simulink model "Discrete_Model"  (R2020b)
settings: Solver=FixedStepAuto  StartTime=0.0  StopTime=3  FixedStep=0.0001  RelTol=1e-3
values from neighbouring files (symbols this model uses):
  B = 3.4    [nonlinear_quicktest.m]
  cont_den = cont_den_master    [nonlinear_quicktest.m]
  cont_den_master = [0.04052 1 0]    [nonlinear_quicktest.m]
  cont_integrator_discrete = discrete_controller(T_sample, disc_type, [0, 1] , [1, 0] )    [nonlinear_quicktest.m]
  cont_num = cont_num_master    [nonlinear_quicktest.m]
  cont_num_master = [1.517, 3.296, 0.2386]    [nonlinear_quicktest.m]
  Delta = 0.0000079    (= 7.9e-06)    [nonlinear_quicktest.m]
  discrete_constants = zeros(2, 2)    [nonlinear_quicktest.m]
  F_lead_param = -1/(alpha_lead_param*T_lead_param)    [nonlinear_quicktest.m]
  G_lead_param = 1    [nonlinear_quicktest.m]
  H_lead_param = k_lead_param/alpha_lead_param*(1/T_lead_param-1/(alpha_lead_param*T_lead_param))    [nonlinear_quicktest.m]
  J_eq = J_1 + n_1^2 *(J_2 + M_3*r_3^2)    (= 2.88733377778e-05)    [nonlinear_quicktest.m]
  k_i = 0.2386    [nonlinear_quicktest.m]
  k_p = 3.296    [nonlinear_quicktest.m]
  K_tau = 42e-3    (= 0.042)    [nonlinear_quicktest.m]
  L_lead_param = k_lead_param/alpha_lead_param    [nonlinear_quicktest.m]
  M_lead_param = 1/L_lead_param    [nonlinear_quicktest.m]    (also in span_optimering_quicker.m = corrections_faktor(i))
  n_1 = 1/3    (= 0.333333333333)    [nonlinear_quicktest.m]
  r_3 = 0.0127    [nonlinear_quicktest.m]
  step_size = step_size_array(j)    [main.m]    (also in nonlinear_quicktest.m = 1; span_optimering_quicker.m = 1)
  T_sample = 0.001    [main.m]    (also in nonlinear_quicktest.m)
  T_t = (k_p/k_i)/10    (= 1.38139145013)    [nonlinear_quicktest.m]
undefined symbols (not defined in the file or in its folder): CoulombAndViscousFriction, CurrentOffset, discrete_controller_pid, j, SignOfVelocity
settings Model: EnablePacing=on  PacingRate=0.001000  Creator=jonas  LastModifiedBy=Bens PC

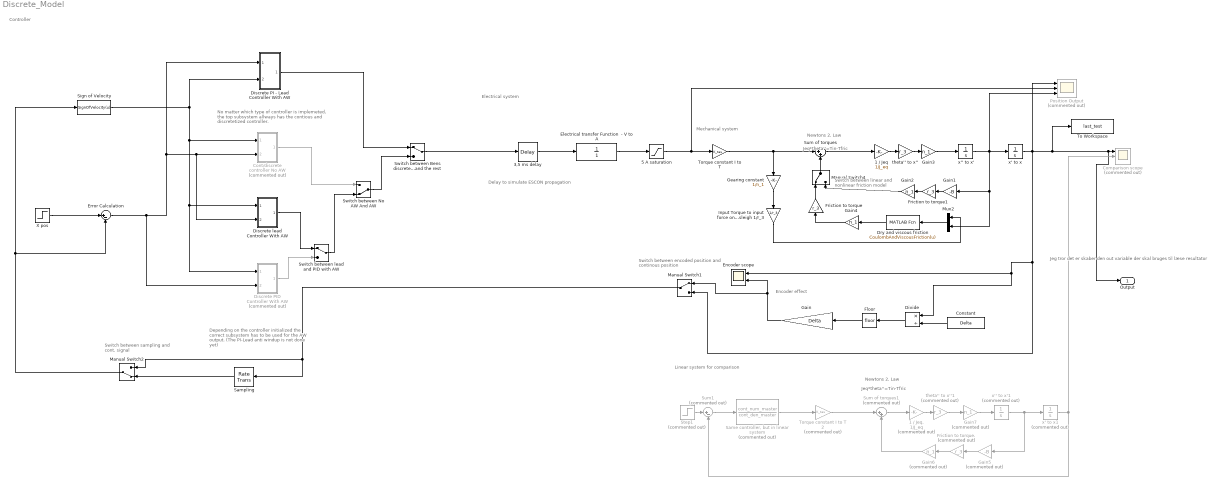
== system Discrete_Model ==
  note: Jeg tror det er skaber den out variable der skal bruges til læse resultator
  note: No matter which type of controller is implemeted,
      | the top subsystem allways has the contious and
      | discretetized controller.
  note: Depending on the controller initialized
      | the correct subsystem has to be used
      | for the AW output. (The PI-Lead anti windup
      | is not done yet)
  note: Controller
  note: Linear system for comparison
  note: Switch between linear
      | and nonlinear friction model
  note: Delay to simulate ESCON propagation
  note: Switch between sampling
      | and cont. signal
  note: Electrical system
  note: Switch between encoded position and
      | continous position
  note: Newtons 2. Law
  note: Mechanical system
  note: Encoder effect
  note: Jeq*theta''=Tin-Tfric
  note: Newtons 2. Law
  note: Jeq*theta''=Tin-Tfric
  1 / Jeq : Gain  Gain=1/J_eq
  1 / Jeq. : Gain  Commented=on  Gain=1/J_eq
  3,5 ms delay : TransportDelay  DelayTime=0.0035
  5 A saturation : Saturate  UpperLimit=5  LowerLimit=-5
  Comparison scope : Scope  Commented=on  NumInputPorts=3
  Constant : Constant  Value=Delta
  Cont/discrete controller No AW : Subsystem  Commented=on
  Discrete PI - Lead Controller With AW : Subsystem
  Discrete PID Controller With AW : Subsystem  Commented=on
  Discrete lead Controller With AW : Subsystem
  Divide : Product  Inputs=*/
  Dry and viscous friction : MATLABFcn  MATLABFcn=CoulombAndViscousFriction(u)  OutputDimensions=1
  Electrical transfer Function  - V to A : TransferFcn  Denominator=[1]
  Encoder scope : Scope  NumInputPorts=2
  Error Calculation : Sum  Inputs=|+-
  Floor : Rounding
  Friction to torque : Gain  Gain=r_3
  Friction to torque. : Gain  Commented=on  Gain=r_3
  Friction to torque1 : Gain  Gain=r_3
  Gain : Gain  Gain=Delta
  Gain1 : Gain  Gain=-B
  Gain2 : Gain  Gain=n_1
  Gain3 : Gain  Gain=n_1
  Gain4 : Gain  Gain=n_1
  Gain5 : Gain  Commented=on  Gain=-B
  Gain6 : Gain  Commented=on  Gain=n_1
  Gain7 : Gain  Commented=on  Gain=n_1
  Gearing constant : Gain  Gain=1/n_1
  Input Torque to input force on sleigh 1/r_3 : Gain  Gain=1/r_3
  Manual Switch1 : ManualSwitch
  Manual Switch2 : ManualSwitch  CurrentSetting=0
  Manual Switch4 : ManualSwitch
  Mux2 : Mux  Inputs=2
  Position Output : Scope  Commented=on  NumInputPorts=3
  "Same controller, but in linear system" : TransferFcn  Commented=on  Numerator=cont_num_master  Denominator=cont_den_master
  "Sampling " : RateTransition  OutPortSampleTime=T_sample
  Sign of Velocity : MATLABFcn  MATLABFcn=SignOfVelocity(u)  OutputDimensions=1
  Step1 : Step  Commented=on  Time=0  After=step_size(j)  SampleTime=0
  Sum of torques : Sum  Inputs=|++
  Sum of torques1 : Sum  Commented=on  Inputs=|++
  Sum1 : Sum  Commented=on  Inputs=|+-
  Switch between Bens discrete PI-Lead AW and the rest : ManualSwitch
  Switch between No AW And AW : ManualSwitch  CurrentSetting=0
  Switch between lead and PID with AW : ManualSwitch
  To Workspace : ToWorkspace  VariableName=last_test  SampleTime=-1
  "Torque constant I to T " : Gain  Gain=K_tau
  Torque constant I to T 2 : Gain  Commented=on  Gain=K_tau
  X pos : Step  Time=0  After=step_size  SampleTime=0
  theta'' to x'' : Gain  Gain=r_3
  theta'' to x''1 : Gain  Commented=on  Gain=r_3
  x' to x : Integrator
  x' to x1 : Integrator  Commented=on
  x'' to x' : Integrator
  x'' to x'1 : Integrator  Commented=on
  Output : Outport
  wires:
  Sum of torques/1 -> 1 / Jeq/1
  theta'' to x''/1 -> Gain3/1
  x'' to x'/1 -> Position Output/3, Gain1/1, Mux2/2, x' to x/1
  Electrical transfer Function  - V to A/1 -> 5 A saturation/1
  Input Torque to input force on sleigh 1/r_3/1 -> Mux2/1
  Mux2/1 -> Dry and viscous friction/1
  5 A saturation/1 -> Position Output/2, "Torque constant I to T "/1
  Gain/1 -> Encoder scope/2, Manual Switch1/1
  Floor/1 -> Gain/1
  Constant/1 -> Divide/2
  Divide/1 -> Floor/1
  Manual Switch1/1 -> "Sampling "/1, Manual Switch2/1
  "Sampling "/1 -> Manual Switch2/2
  Dry and viscous friction/1 -> Gain4/1
  3,5 ms delay/1 -> Electrical transfer Function  - V to A/1
  1 / Jeq/1 -> theta'' to x''/1
  Manual Switch4/1 -> Sum of torques/2
  Friction to torque/1 -> Manual Switch4/1
  Gain1/1 -> Friction to torque1/1
  Friction to torque1/1 -> Gain2/1
  "Torque constant I to T "/1 -> Sum of torques/1, Gearing constant/1
  Gearing constant/1 -> Input Torque to input force on sleigh 1/r_3/1
  Gain2/1 -> Manual Switch4/2
  Gain3/1 -> x'' to x'/1
  Gain4/1 -> Friction to torque/1
  Friction to torque./1 -> Gain6/1
  Gain7/1 -> x'' to x'1/1
  Gain5/1 -> Friction to torque./1
  x'' to x'1/1 -> Gain5/1, x' to x1/1
  Gain6/1 -> Sum of torques1/2
  1 / Jeq./1 -> theta'' to x''1/1
  Sum of torques1/1 -> 1 / Jeq./1
  Sum1/1 -> "Same controller, but in linear system"/1
  Step1/1 -> Sum1/1
  Torque constant I to T 2/1 -> Sum of torques1/1
  x' to x/1 -> Position Output/1, To Workspace/1, Output/1, Comparison scope/1, Divide/1, Encoder scope/1, Manual Switch1/2
  x' to x1/1 -> Comparison scope/2, Sum1/2
  "Same controller, but in linear system"/1 -> Torque constant I to T 2/1
  theta'' to x''1/1 -> Gain7/1
  Sign of Velocity/1 -> Discrete PI - Lead Controller With AW/2(Sign of velocity in), Discrete PID Controller With AW/1(In1), Discrete lead Controller With AW/1(Sign of velocity in), Cont/discrete controller No AW/1(In1)
  Cont/discrete controller No AW/1(Out1) -> Switch between No AW And AW/1
  Discrete lead Controller With AW/1(Out1) -> Switch between lead and PID with AW/1
  Discrete PID Controller With AW/1(Out1) -> Switch between lead and PID with AW/2
  Switch between lead and PID with AW/1 -> Switch between No AW And AW/2
  Manual Switch2/1 -> Sign of Velocity/1, Error Calculation/2
  Discrete PI - Lead Controller With AW/1(Out3) -> Switch between Bens discrete PI-Lead AW and the rest/1
  Switch between No AW And AW/1 -> Switch between Bens discrete PI-Lead AW and the rest/2
  Switch between Bens discrete PI-Lead AW and the rest/1 -> 3,5 ms delay/1
  X pos/1 -> Error Calculation/1
  Error Calculation/1 -> Discrete PID Controller With AW/2(In2), Discrete PI - Lead Controller With AW/1(Error in), Discrete lead Controller With AW/2(Error in), Cont/discrete controller No AW/2(In2)

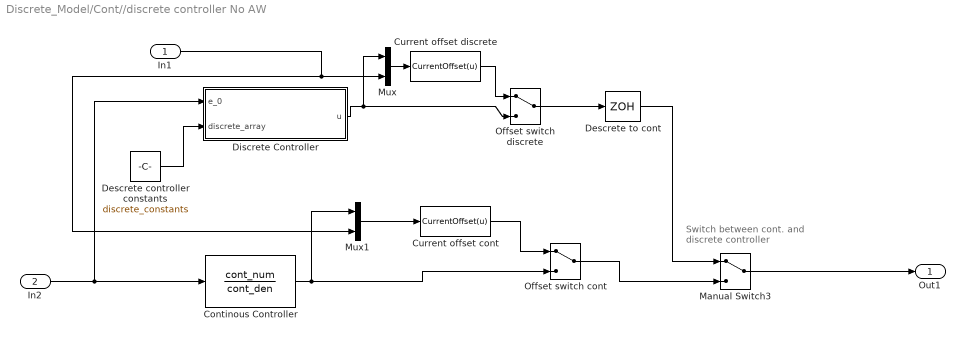
== system Discrete_Model/Cont//discrete controller No AW ==
  note: Switch between cont.
      | and discrete controller
  In1 : Inport
  In2 : Inport  Port=2
  Continous Controller : TransferFcn  Numerator=cont_num  Denominator=cont_den
  Current offset cont : MATLABFcn  MATLABFcn=CurrentOffset(u)  OutputDimensions=1
  Current offset discrete : MATLABFcn  MATLABFcn=CurrentOffset(u)  OutputDimensions=1
  Descrete controller constants : Constant  Value=discrete_constants
  Descrete to cont : ZeroOrderHold  SampleTime=T_sample
  Discrete Controller : MATLAB Function  TreatAsAtomicUnit=on
  Manual Switch3 : ManualSwitch
  Mux : Mux  Inputs=2
  Mux1 : Mux  Inputs=2
  Offset switch cont : ManualSwitch
  Offset switch discrete : ManualSwitch
  Out1 : Outport
  wires:
  Manual Switch3/1 -> Out1/1
  In1/1 -> Mux/2, Mux1/2
  In2/1 -> Continous Controller/1, Discrete Controller/1(e_0)
  Current offset discrete/1 -> Offset switch discrete/1
  Descrete to cont/1 -> Manual Switch3/1
  Offset switch discrete/1 -> Descrete to cont/1
  Offset switch cont/1 -> Manual Switch3/2
  Discrete Controller/1(u) -> Offset switch discrete/2, Mux/1
  Mux/1 -> Current offset discrete/1
  Descrete controller constants/1 -> Discrete Controller/2(discrete_array)
  Mux1/1 -> Current offset cont/1
  Continous Controller/1 -> Mux1/1, Offset switch cont/2
  Current offset cont/1 -> Offset switch cont/1

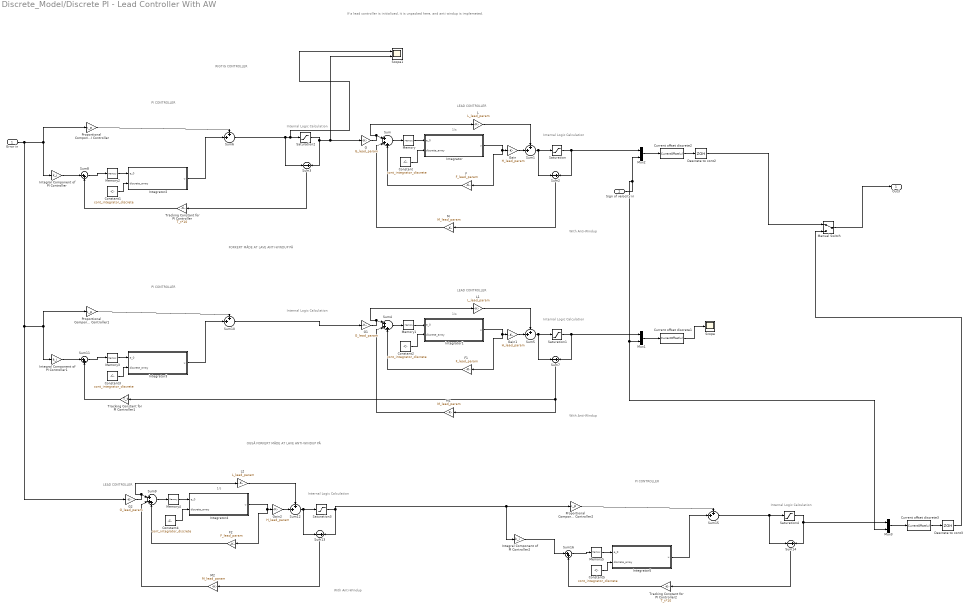
== system Discrete_Model/Discrete PI - Lead Controller With AW ==
  note: RIGTIG CONTROLLER
  note: Internal Logic Calculation
  note: LEAD CONTROLLER
  note: With Anti-Windup
  note: 1/s
  note: If a lead controller is initialized, it is unpacked here, and anti windup is implemeted.
  note: PI CONTROLLER
  note: Internal Logic Calculation
  note: Internal Logic Calculation
  note: LEAD CONTROLLER
  note: With Anti-Windup
  note: 1/s
  note: PI CONTROLLER
  note: Internal Logic Calculation
  note: Internal Logic Calculation
  note: LEAD CONTROLLER
  note: With Anti-Windup
  note: 1/s
  note: PI CONTROLLER
  note: Internal Logic Calculation
  note: FORKERT MÅDE AT LAVE ANTI-WINDUP PÅ
  note: OGSÅ FORKERT MÅDE AT LAVE ANTI-WINDUP PÅ
  Error in : Inport
  Sign of velocity in : Inport  Port=2
  Constant{,1..5} (6 alike) : Constant  Value=cont_integrator_discrete
  Current offset discrete1 : MATLABFcn  MATLABFcn=CurrentOffset(u)  OutputDimensions=1
  Current offset discrete2 : MATLABFcn  MATLABFcn=CurrentOffset(u)  OutputDimensions=1
  Current offset discrete3 : MATLABFcn  MATLABFcn=CurrentOffset(u)  OutputDimensions=1
  Descrete to cont2 : ZeroOrderHold  SampleTime=T_sample
  Descrete to cont3 : ZeroOrderHold  SampleTime=T_sample
  F : Gain  Gain=F_lead_param
  F1 : Gain  Gain=F_lead_param
  F2 : Gain  Gain=F_lead_param
  G : Gain  Gain=G_lead_param
  G1 : Gain  Gain=G_lead_param
  G2 : Gain  Gain=G_lead_param
  Gain : Gain  Gain=H_lead_param
  Gain1 : Gain  Gain=H_lead_param
  Gain2 : Gain  Gain=H_lead_param
  Integral Component of PI Controller : Gain  Gain=k_i
  Integral Component of PI Controller1 : Gain  Gain=k_i
  Integral Component of PI Controller2 : Gain  Gain=k_i
  Integrator : MATLAB Function  TreatAsAtomicUnit=on
  Integrator1 : MATLAB Function  TreatAsAtomicUnit=on
  Integrator2 : MATLAB Function  TreatAsAtomicUnit=on
  Integrator3 : MATLAB Function  TreatAsAtomicUnit=on
  Integrator4 : MATLAB Function  TreatAsAtomicUnit=on
  Integrator5 : MATLAB Function  TreatAsAtomicUnit=on
  L : Gain  Gain=L_lead_param
  L1 : Gain  Gain=L_lead_param
  L2 : Gain  Gain=L_lead_param
  M : Gain  Gain=M_lead_param
  M1 : Gain  Gain=M_lead_param
  M2 : Gain  Gain=M_lead_param
  Manual Switch : ManualSwitch
  Memory{,1..5} (6 alike) : Memory
  Mux1 : Mux  Inputs=2
  Mux2 : Mux  Inputs=2
  Mux3 : Mux  Inputs=2
  Proportional Component of PI Controller : Gain  Gain=k_p
  Proportional Component of PI Controller1 : Gain  Gain=k_p
  Proportional Component of PI Controller2 : Gain  Gain=k_p
  Saturation{,1..4} (5 alike) : Saturate  UpperLimit=5  LowerLimit=-5
  Scope : Scope
  Scope1 : Scope  NumInputPorts=2
  Sum : Sum  Inputs=|+++
  Sum{1,5..6,10,12,15} (6 alike) : Sum  Inputs=++|
  Sum11 : Sum  Inputs=|++
  Sum{2..3,7,13..14} (5 alike) : Sum  Inputs=-+
  Sum16 : Sum  Inputs=|++
  Sum4 : Sum  Inputs=|+++
  Sum8 : Sum  Inputs=|++
  Sum9 : Sum  Inputs=|+++
  Tracking Constant for PI Controller : Gain  Gain=T_t*10
  Tracking Constant for PI Controller1 : Gain  Gain=T_t
  Tracking Constant for PI Controller2 : Gain  Gain=T_t*10
  Out3 : Outport
  wires:
  Mux2/1 -> Current offset discrete2/1
  Current offset discrete2/1 -> Descrete to cont2/1
  Sign of velocity in/1 -> Mux3/2, Mux1/2, Mux2/2
  Sum/1 -> Memory/1
  Memory/1 -> Integrator/1(e_0)
  Saturation/1 -> Mux2/1, Sum2/2
  Constant/1 -> Integrator/2(discrete_array)
  Sum2/1 -> M/1
  M/1 -> Sum/2
  L/1 -> Sum1/1
  Sum1/1 -> Saturation/1, Sum2/1
  G/1 -> L/1, Sum/1
  Integrator/1(u) -> F/1, Gain/1
  F/1 -> Sum/3
  Gain/1 -> Sum1/2
  Saturation2/1 -> Sum3/2, Scope1/2, G/1
  Memory2/1 -> Integrator2/1(e_0)
  Integral Component of PI Controller/1 -> Sum8/1
  Sum8/1 -> Memory2/1
  Constant1/1 -> Integrator2/2(discrete_array)
  Proportional Component of PI Controller/1 -> Sum6/1
  Tracking Constant for PI Controller/1 -> Sum8/2
  Integrator2/1(u) -> Sum6/2
  Sum6/1 -> Scope1/1, Saturation2/1, Sum3/1
  Sum3/1 -> Tracking Constant for PI Controller/1
  Sum7/1 -> M1/1, Tracking Constant for PI Controller1/1
  Integrator3/1(u) -> Sum10/2
  Tracking Constant for PI Controller1/1 -> Sum11/2
  Proportional Component of PI Controller1/1 -> Sum10/1
  Constant3/1 -> Integrator3/2(discrete_array)
  Sum11/1 -> Memory3/1
  Integral Component of PI Controller1/1 -> Sum11/1
  Memory3/1 -> Integrator3/1(e_0)
  Sum10/1 -> G1/1
  Error in/1 -> Proportional Component of PI Controller/1, Integral Component of PI Controller/1, G2/1, Integral Component of PI Controller1/1, Proportional Component of PI Controller1/1
  Gain1/1 -> Sum5/2
  F1/1 -> Sum4/3
  Integrator1/1(u) -> Gain1/1, F1/1
  G1/1 -> Sum4/1, L1/1
  Sum5/1 -> Sum7/1, Saturation1/1
  L1/1 -> Sum5/1
  M1/1 -> Sum4/2
  Constant2/1 -> Integrator1/2(discrete_array)
  Saturation1/1 -> Sum7/2, Mux1/1
  Memory1/1 -> Integrator1/1(e_0)
  Sum4/1 -> Memory1/1
  Mux1/1 -> Current offset discrete1/1
  Descrete to cont2/1 -> Manual Switch/1
  Manual Switch/1 -> Out3/1
  Saturation3/1 -> Integral Component of PI Controller2/1, Proportional Component of PI Controller2/1, Sum13/2
  Sum14/1 -> Tracking Constant for PI Controller2/1
  Sum15/1 -> Sum14/1, Saturation4/1
  Integrator5/1(u) -> Sum15/2
  Tracking Constant for PI Controller2/1 -> Sum16/2
  Proportional Component of PI Controller2/1 -> Sum15/1
  Constant5/1 -> Integrator5/2(discrete_array)
  Sum16/1 -> Memory5/1
  Integral Component of PI Controller2/1 -> Sum16/1
  Memory5/1 -> Integrator5/1(e_0)
  Saturation4/1 -> Mux3/1, Sum14/2
  Gain2/1 -> Sum12/2
  F2/1 -> Sum9/3
  Integrator4/1(u) -> Gain2/1, F2/1
  G2/1 -> Sum9/1, L2/1
  Sum12/1 -> Sum13/1, Saturation3/1
  L2/1 -> Sum12/1
  M2/1 -> Sum9/2
  Sum13/1 -> M2/1
  Constant4/1 -> Integrator4/2(discrete_array)
  Memory4/1 -> Integrator4/1(e_0)
  Sum9/1 -> Memory4/1
  Current offset discrete3/1 -> Descrete to cont3/1
  Mux3/1 -> Current offset discrete3/1
  Descrete to cont3/1 -> Manual Switch/2
  Current offset discrete1/1 -> Scope/1

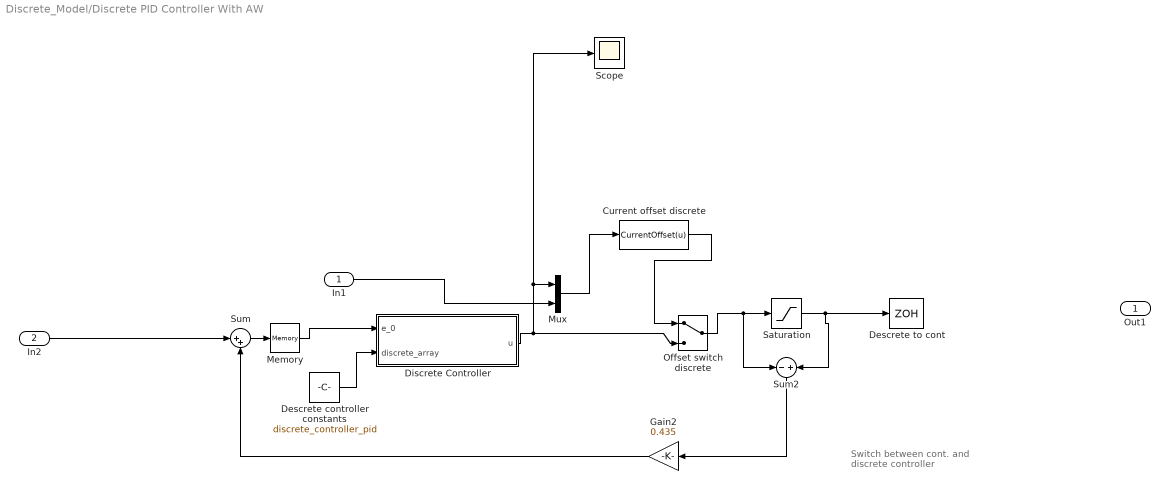
== system Discrete_Model/Discrete PID Controller With AW ==
  note: Switch between cont.
      | and discrete controller
  In1 : Inport
  In2 : Inport  Port=2
  Current offset discrete : MATLABFcn  MATLABFcn=CurrentOffset(u)  OutputDimensions=1
  Descrete controller constants : Constant  Value=discrete_controller_pid
  Descrete to cont : ZeroOrderHold  SampleTime=T_sample
  Discrete Controller : MATLAB Function  TreatAsAtomicUnit=on
  Gain2 : Gain  Gain=0.435
  Memory : Memory
  Mux : Mux  Inputs=3
  Offset switch discrete : ManualSwitch
  Saturation : Saturate
  Scope : Scope
  Sum : Sum  Inputs=|++
  Sum2 : Sum  Inputs=-+
  Out1 : Outport
  wires:
  In1/1 -> Mux/3
  Mux/1 -> Current offset discrete/1
  Descrete controller constants/1 -> Discrete Controller/2(discrete_array)
  Discrete Controller/1(u) -> Offset switch discrete/2, Scope/1, Mux/1
  Current offset discrete/1 -> Offset switch discrete/1
  ? -> Out1/1
  In2/1 -> Sum/1
  Sum2/1 -> Gain2/1
  Gain2/1 -> Sum/2
  Offset switch discrete/1 -> Sum2/1, Saturation/1
  Saturation/1 -> Sum2/2, Descrete to cont/1
  Sum/1 -> Memory/1
  Memory/1 -> Discrete Controller/1(e_0)

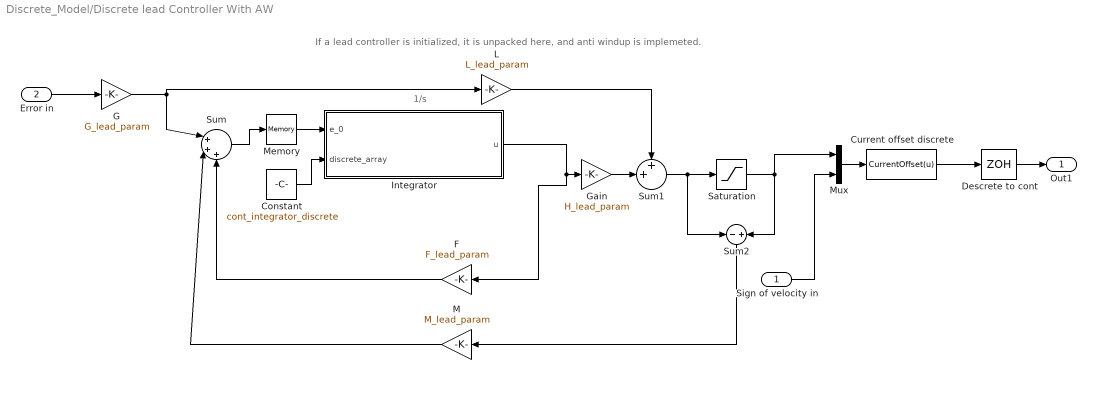
== system Discrete_Model/Discrete lead Controller With AW ==
  note: 1/s
  note: If a lead controller is initialized, it is unpacked here, and anti windup is implemeted.
  Sign of velocity in : Inport
  Error in : Inport  Port=2
  Constant : Constant  Value=cont_integrator_discrete
  Current offset discrete : MATLABFcn  MATLABFcn=CurrentOffset(u)  OutputDimensions=1
  Descrete to cont : ZeroOrderHold  SampleTime=T_sample
  F : Gain  Gain=F_lead_param
  G : Gain  Gain=G_lead_param
  Gain : Gain  Gain=H_lead_param
  Integrator : MATLAB Function  TreatAsAtomicUnit=on
  L : Gain  Gain=L_lead_param
  M : Gain  Gain=M_lead_param
  Memory : Memory
  Mux : Mux  Inputs=2
  Saturation : Saturate  UpperLimit=5  LowerLimit=-5
  Sum : Sum  Inputs=|+++
  Sum1 : Sum  Inputs=++|
  Sum2 : Sum  Inputs=-+
  Out1 : Outport
  wires:
  Mux/1 -> Current offset discrete/1
  Sign of velocity in/1 -> Mux/2
  Current offset discrete/1 -> Descrete to cont/1
  Descrete to cont/1 -> Out1/1
  Error in/1 -> G/1
  Integrator/1(u) -> F/1, Gain/1
  G/1 -> Sum/1, L/1
  F/1 -> Sum/3
  Sum/1 -> Memory/1
  Gain/1 -> Sum1/2
  L/1 -> Sum1/1
  Sum1/1 -> Sum2/1, Saturation/1
  Saturation/1 -> Mux/1, Sum2/2
  Sum2/1 -> M/1
  M/1 -> Sum/2
  Constant/1 -> Integrator/2(discrete_array)
  Memory/1 -> Integrator/1(e_0)

== matlab function Discrete_Model/Discrete lead Controller With AW/Integrator ==
  settings: updateMethod=DISCRETE  sampleTime=T_sample
  data: e_0 input; u output; discrete_array input
function u = Controller(e_0, discrete_array)
persistent u_1 e_1 e_2 e_3 e_4 u_2 u_3 u_4 ;

coder.extrinsic('evalin', 'assignin') %% this allows access to T_sample
T = 0;
T = evalin('base','T_sample'); % Read value from workspace



%% discrete array input has the following format
%discrete_array(1) =  u_n FD array 
%discrete_array(2) =  e_n FD array 
%discrete_array(3) =  u_n BD array 
%discrete_array(4) =  e_n BD array 




%% With a FD controller
u_n_array = discrete_array(3, 1:end);
e_n_array = discrete_array(4, 1:end);











% Continuous controller : 
%tf_numerator = [1.203 3.6];
%tf_denomenator = [0.04812 1];




%Discrete output from program














if isempty(e_1)
    e_1 = 0;
end
if isempty(e_2)
    e_2 = 0;
end
if isempty(e_3)
    e_3 = 0;
end
if isempty(u_1)
    u_1 = 0;
end

if isempty(u_2)
    u_2 = 0;
end
if isempty(u_3)
    u_3 = 0;
end
if isempty(e_4)
    e_4 = 0;
end
if isempty(u_4)
    u_4 = 0;
end





e_n_length = length(e_n_array);
u_n_length = length(u_n_array); 

if e_n_length == 1
    e_n_equation = e_0 * e_n_array(1);
elseif e_n_length ==2
        e_n_equation = e_0 * e_n_array(1) + e_1 * e_n_array(2);
elseif e_n_length ==3
        e_n_equation = e_0 * e_n_array(1) + e_n_array(2) * e_1 + e_2 * e_n_array(3);
elseif e_n_length ==4
        e_n_equation = e_0 * e_n_array(1) + e_n_array(2) * e_1 + e_2 * e_n_array(3) + e_3 * e_n_array(4);
else
    e_n_equation = 0
end

if u_n_length == 1
        u_n_equation = u_1 * u_n_array(1);
elseif u_n_length == 2
        u_n_equation = u_1 * u_n_array(1) + u_2 * u_n_array(2);
elseif u_n_length ==3
        u_n_equation = u_1 * u_n_array(1) + u_n_array(2) * u_2 + u_3 * u_n_array(3);
elseif u_n_length ==4
        u_n_equation = u_1 * u_n_array(1) + u_n_array(2) * u_2 + u_3 * u_n_array(3) + u_4 * u_n_array(4);
else
    u_n_equation = 0;
end



u = e_n_equation + u_n_equation;

e_3 = e_2;
e_2=e_1;
e_1=e_0;

u_4 = u_3;
u_3 = u_2;
u_2 = u_1;

u_1=u;

end

== matlab function Discrete_Model/Discrete PID Controller With AW/Discrete Controller ==
  settings: updateMethod=DISCRETE  sampleTime=T_sample
  data: e_0 input; u output; discrete_array input
function u = Controller(e_0, discrete_array)
persistent u_1 e_1 e_2 e_3 e_4 u_2 u_3 u_4 ;

coder.extrinsic('evalin', 'assignin') %% this allows access to T_sample
T = 0;
T = evalin('base','T_sample'); % Read value from workspace



%% discrete array input has the following format
%discrete_array(1) =  u_n FD array 
%discrete_array(2) =  e_n FD array 
%discrete_array(3) =  u_n BD array 
%discrete_array(4) =  e_n BD array 



%% With a FD controller
u_n_array = discrete_array(1, 1:end);
e_n_array = discrete_array(2, 1:end);











% Continuous controller : 
%tf_numerator = [1.203 3.6];
%tf_denomenator = [0.04812 1];




%Discrete output from program














if isempty(e_1)
    e_1 = 0;
end
if isempty(e_2)
    e_2 = 0;
end
if isempty(e_3)
    e_3 = 0;
end
if isempty(u_1)
    u_1 = 0;
end

if isempty(u_2)
    u_2 = 0;
end
if isempty(u_3)
    u_3 = 0;
end
if isempty(e_4)
    e_4 = 0;
end
if isempty(u_4)
    u_4 = 0;
end





e_n_length = length(e_n_array);
u_n_length = length(u_n_array); 

if e_n_length == 1
    e_n_equation = e_0 * e_n_array(1);
elseif e_n_length ==2
        e_n_equation = e_0 * e_n_array(1) + e_1 * e_n_array(2);
elseif e_n_length ==3
        e_n_equation = e_0 * e_n_array(1) + e_n_array(2) * e_1 + e_2 * e_n_array(3);
elseif e_n_length ==4
        e_n_equation = e_0 * e_n_array(1) + e_n_array(2) * e_1 + e_2 * e_n_array(3) + e_3 * e_n_array(4);
else
    e_n_equation = 0
end

if u_n_length == 1
        u_n_equation = u_1 * u_n_array(1);
elseif u_n_length == 2
        u_n_equation = u_1 * u_n_array(1) + u_2 * u_n_array(2);
elseif u_n_length ==3
        u_n_equation = u_1 * u_n_array(1) + u_n_array(2) * u_2 + u_3 * u_n_array(3);
elseif u_n_length ==4
        u_n_equation = u_1 * u_n_array(1) + u_n_array(2) * u_2 + u_3 * u_n_array(3) + u_4 * u_n_array(4);
else
    u_n_equation = 0;
end



u = e_n_equation + u_n_equation;

%u = (1447209*e_2 + 1203000*T*u_1 - e_1*(30075000*T + 2894418) + e_0*(90000000*T^2 + 30075000*T + 1447209))/(1000*T*(25000*T + 1203));

e_3 = e_2;
e_2=e_1;
e_1=e_0;

u_4 = u_3;
u_3 = u_2;
u_2 = u_1;

u_1=u;

end

== matlab function Discrete_Model/Discrete PI - Lead Controller With AW/Integrator1 ==
  settings: updateMethod=DISCRETE  sampleTime=T_sample
  data: e_0 input; u output; discrete_array input
function u = Controller(e_0, discrete_array)
persistent u_1 e_1 e_2 e_3 e_4 u_2 u_3 u_4 ;

coder.extrinsic('evalin', 'assignin') %% this allows access to T_sample
T = 0;
T = evalin('base','T_sample'); % Read value from workspace



%% discrete array input has the following format
%discrete_array(1) =  u_n FD array 
%discrete_array(2) =  e_n FD array 
%discrete_array(3) =  u_n BD array 
%discrete_array(4) =  e_n BD array 




%% With a FD controller
u_n_array = discrete_array(3, 1:end);
e_n_array = discrete_array(4, 1:end);











% Continuous controller : 
%tf_numerator = [1.203 3.6];
%tf_denomenator = [0.04812 1];




%Discrete output from program














if isempty(e_1)
    e_1 = 0;
end
if isempty(e_2)
    e_2 = 0;
end
if isempty(e_3)
    e_3 = 0;
end
if isempty(u_1)
    u_1 = 0;
end

if isempty(u_2)
    u_2 = 0;
end
if isempty(u_3)
    u_3 = 0;
end
if isempty(e_4)
    e_4 = 0;
end
if isempty(u_4)
    u_4 = 0;
end





e_n_length = length(e_n_array);
u_n_length = length(u_n_array); 

if e_n_length == 1
    e_n_equation = e_0 * e_n_array(1);
elseif e_n_length ==2
        e_n_equation = e_0 * e_n_array(1) + e_1 * e_n_array(2);
elseif e_n_length ==3
        e_n_equation = e_0 * e_n_array(1) + e_n_array(2) * e_1 + e_2 * e_n_array(3);
elseif e_n_length ==4
        e_n_equation = e_0 * e_n_array(1) + e_n_array(2) * e_1 + e_2 * e_n_array(3) + e_3 * e_n_array(4);
else
    e_n_equation = 0
end

if u_n_length == 1
        u_n_equation = u_1 * u_n_array(1);
elseif u_n_length == 2
        u_n_equation = u_1 * u_n_array(1) + u_2 * u_n_array(2);
elseif u_n_length ==3
        u_n_equation = u_1 * u_n_array(1) + u_n_array(2) * u_2 + u_3 * u_n_array(3);
elseif u_n_length ==4
        u_n_equation = u_1 * u_n_array(1) + u_n_array(2) * u_2 + u_3 * u_n_array(3) + u_4 * u_n_array(4);
else
    u_n_equation = 0;
end



u = e_n_equation + u_n_equation;

e_3 = e_2;
e_2=e_1;
e_1=e_0;

u_4 = u_3;
u_3 = u_2;
u_2 = u_1;

u_1=u;

end

== matlab function Discrete_Model/Discrete PI - Lead Controller With AW/Integrator3 ==
  settings: updateMethod=DISCRETE  sampleTime=T_sample
  data: e_0 input; u output; discrete_array input
function u = Controller(e_0, discrete_array)
persistent u_1 e_1 e_2 e_3 e_4 u_2 u_3 u_4 ;

coder.extrinsic('evalin', 'assignin') %% this allows access to T_sample
T = 0;
T = evalin('base','T_sample'); % Read value from workspace



%% discrete array input has the following format
%discrete_array(1) =  u_n FD array 
%discrete_array(2) =  e_n FD array 
%discrete_array(3) =  u_n BD array 
%discrete_array(4) =  e_n BD array 




%% With a FD controller
u_n_array = discrete_array(3, 1:end);
e_n_array = discrete_array(4, 1:end);











% Continuous controller : 
%tf_numerator = [1.203 3.6];
%tf_denomenator = [0.04812 1];




%Discrete output from program














if isempty(e_1)
    e_1 = 0;
end
if isempty(e_2)
    e_2 = 0;
end
if isempty(e_3)
    e_3 = 0;
end
if isempty(u_1)
    u_1 = 0;
end

if isempty(u_2)
    u_2 = 0;
end
if isempty(u_3)
    u_3 = 0;
end
if isempty(e_4)
    e_4 = 0;
end
if isempty(u_4)
    u_4 = 0;
end





e_n_length = length(e_n_array);
u_n_length = length(u_n_array); 

if e_n_length == 1
    e_n_equation = e_0 * e_n_array(1);
elseif e_n_length ==2
        e_n_equation = e_0 * e_n_array(1) + e_1 * e_n_array(2);
elseif e_n_length ==3
        e_n_equation = e_0 * e_n_array(1) + e_n_array(2) * e_1 + e_2 * e_n_array(3);
elseif e_n_length ==4
        e_n_equation = e_0 * e_n_array(1) + e_n_array(2) * e_1 + e_2 * e_n_array(3) + e_3 * e_n_array(4);
else
    e_n_equation = 0
end

if u_n_length == 1
        u_n_equation = u_1 * u_n_array(1);
elseif u_n_length == 2
        u_n_equation = u_1 * u_n_array(1) + u_2 * u_n_array(2);
elseif u_n_length ==3
        u_n_equation = u_1 * u_n_array(1) + u_n_array(2) * u_2 + u_3 * u_n_array(3);
elseif u_n_length ==4
        u_n_equation = u_1 * u_n_array(1) + u_n_array(2) * u_2 + u_3 * u_n_array(3) + u_4 * u_n_array(4);
else
    u_n_equation = 0;
end



u = e_n_equation + u_n_equation;

e_3 = e_2;
e_2=e_1;
e_1=e_0;

u_4 = u_3;
u_3 = u_2;
u_2 = u_1;

u_1=u;

end

== matlab function Discrete_Model/Discrete PI - Lead Controller With AW/Integrator ==
  settings: updateMethod=DISCRETE  sampleTime=T_sample
  data: e_0 input; u output; discrete_array input
function u = Controller(e_0, discrete_array)
persistent u_1 e_1 e_2 e_3 e_4 u_2 u_3 u_4 ;

coder.extrinsic('evalin', 'assignin') %% this allows access to T_sample
T = 0;
T = evalin('base','T_sample'); % Read value from workspace



%% discrete array input has the following format
%discrete_array(1) =  u_n FD array 
%discrete_array(2) =  e_n FD array 
%discrete_array(3) =  u_n BD array 
%discrete_array(4) =  e_n BD array 




%% With a FD controller
u_n_array = discrete_array(3, 1:end);
e_n_array = discrete_array(4, 1:end);











% Continuous controller : 
%tf_numerator = [1.203 3.6];
%tf_denomenator = [0.04812 1];




%Discrete output from program














if isempty(e_1)
    e_1 = 0;
end
if isempty(e_2)
    e_2 = 0;
end
if isempty(e_3)
    e_3 = 0;
end
if isempty(u_1)
    u_1 = 0;
end

if isempty(u_2)
    u_2 = 0;
end
if isempty(u_3)
    u_3 = 0;
end
if isempty(e_4)
    e_4 = 0;
end
if isempty(u_4)
    u_4 = 0;
end





e_n_length = length(e_n_array);
u_n_length = length(u_n_array); 

if e_n_length == 1
    e_n_equation = e_0 * e_n_array(1);
elseif e_n_length ==2
        e_n_equation = e_0 * e_n_array(1) + e_1 * e_n_array(2);
elseif e_n_length ==3
        e_n_equation = e_0 * e_n_array(1) + e_n_array(2) * e_1 + e_2 * e_n_array(3);
elseif e_n_length ==4
        e_n_equation = e_0 * e_n_array(1) + e_n_array(2) * e_1 + e_2 * e_n_array(3) + e_3 * e_n_array(4);
else
    e_n_equation = 0
end

if u_n_length == 1
        u_n_equation = u_1 * u_n_array(1);
elseif u_n_length == 2
        u_n_equation = u_1 * u_n_array(1) + u_2 * u_n_array(2);
elseif u_n_length ==3
        u_n_equation = u_1 * u_n_array(1) + u_n_array(2) * u_2 + u_3 * u_n_array(3);
elseif u_n_length ==4
        u_n_equation = u_1 * u_n_array(1) + u_n_array(2) * u_2 + u_3 * u_n_array(3) + u_4 * u_n_array(4);
else
    u_n_equation = 0;
end



u = e_n_equation + u_n_equation;

e_3 = e_2;
e_2=e_1;
e_1=e_0;

u_4 = u_3;
u_3 = u_2;
u_2 = u_1;

u_1=u;

end

== matlab function Discrete_Model/Discrete PI - Lead Controller With AW/Integrator4 ==
  settings: updateMethod=DISCRETE  sampleTime=T_sample
  data: e_0 input; u output; discrete_array input
function u = Controller(e_0, discrete_array)
persistent u_1 e_1 e_2 e_3 e_4 u_2 u_3 u_4 ;

coder.extrinsic('evalin', 'assignin') %% this allows access to T_sample
T = 0;
T = evalin('base','T_sample'); % Read value from workspace



%% discrete array input has the following format
%discrete_array(1) =  u_n FD array 
%discrete_array(2) =  e_n FD array 
%discrete_array(3) =  u_n BD array 
%discrete_array(4) =  e_n BD array 




%% With a FD controller
u_n_array = discrete_array(3, 1:end);
e_n_array = discrete_array(4, 1:end);











% Continuous controller : 
%tf_numerator = [1.203 3.6];
%tf_denomenator = [0.04812 1];




%Discrete output from program














if isempty(e_1)
    e_1 = 0;
end
if isempty(e_2)
    e_2 = 0;
end
if isempty(e_3)
    e_3 = 0;
end
if isempty(u_1)
    u_1 = 0;
end

if isempty(u_2)
    u_2 = 0;
end
if isempty(u_3)
    u_3 = 0;
end
if isempty(e_4)
    e_4 = 0;
end
if isempty(u_4)
    u_4 = 0;
end





e_n_length = length(e_n_array);
u_n_length = length(u_n_array); 

if e_n_length == 1
    e_n_equation = e_0 * e_n_array(1);
elseif e_n_length ==2
        e_n_equation = e_0 * e_n_array(1) + e_1 * e_n_array(2);
elseif e_n_length ==3
        e_n_equation = e_0 * e_n_array(1) + e_n_array(2) * e_1 + e_2 * e_n_array(3);
elseif e_n_length ==4
        e_n_equation = e_0 * e_n_array(1) + e_n_array(2) * e_1 + e_2 * e_n_array(3) + e_3 * e_n_array(4);
else
    e_n_equation = 0
end

if u_n_length == 1
        u_n_equation = u_1 * u_n_array(1);
elseif u_n_length == 2
        u_n_equation = u_1 * u_n_array(1) + u_2 * u_n_array(2);
elseif u_n_length ==3
        u_n_equation = u_1 * u_n_array(1) + u_n_array(2) * u_2 + u_3 * u_n_array(3);
elseif u_n_length ==4
        u_n_equation = u_1 * u_n_array(1) + u_n_array(2) * u_2 + u_3 * u_n_array(3) + u_4 * u_n_array(4);
else
    u_n_equation = 0;
end



u = e_n_equation + u_n_equation;

e_3 = e_2;
e_2=e_1;
e_1=e_0;

u_4 = u_3;
u_3 = u_2;
u_2 = u_1;

u_1=u;

end

== matlab function Discrete_Model/Discrete PI - Lead Controller With AW/Integrator5 ==
  settings: updateMethod=DISCRETE  sampleTime=T_sample
  data: e_0 input; u output; discrete_array input
function u = Controller(e_0, discrete_array)
persistent u_1 e_1 e_2 e_3 e_4 u_2 u_3 u_4 ;

coder.extrinsic('evalin', 'assignin') %% this allows access to T_sample
T = 0;
T = evalin('base','T_sample'); % Read value from workspace



%% discrete array input has the following format
%discrete_array(1) =  u_n FD array 
%discrete_array(2) =  e_n FD array 
%discrete_array(3) =  u_n BD array 
%discrete_array(4) =  e_n BD array 




%% With a FD controller
u_n_array = discrete_array(3, 1:end);
e_n_array = discrete_array(4, 1:end);











% Continuous controller : 
%tf_numerator = [1.203 3.6];
%tf_denomenator = [0.04812 1];




%Discrete output from program














if isempty(e_1)
    e_1 = 0;
end
if isempty(e_2)
    e_2 = 0;
end
if isempty(e_3)
    e_3 = 0;
end
if isempty(u_1)
    u_1 = 0;
end

if isempty(u_2)
    u_2 = 0;
end
if isempty(u_3)
    u_3 = 0;
end
if isempty(e_4)
    e_4 = 0;
end
if isempty(u_4)
    u_4 = 0;
end





e_n_length = length(e_n_array);
u_n_length = length(u_n_array); 

if e_n_length == 1
    e_n_equation = e_0 * e_n_array(1);
elseif e_n_length ==2
        e_n_equation = e_0 * e_n_array(1) + e_1 * e_n_array(2);
elseif e_n_length ==3
        e_n_equation = e_0 * e_n_array(1) + e_n_array(2) * e_1 + e_2 * e_n_array(3);
elseif e_n_length ==4
        e_n_equation = e_0 * e_n_array(1) + e_n_array(2) * e_1 + e_2 * e_n_array(3) + e_3 * e_n_array(4);
else
    e_n_equation = 0
end

if u_n_length == 1
        u_n_equation = u_1 * u_n_array(1);
elseif u_n_length == 2
        u_n_equation = u_1 * u_n_array(1) + u_2 * u_n_array(2);
elseif u_n_length ==3
        u_n_equation = u_1 * u_n_array(1) + u_n_array(2) * u_2 + u_3 * u_n_array(3);
elseif u_n_length ==4
        u_n_equation = u_1 * u_n_array(1) + u_n_array(2) * u_2 + u_3 * u_n_array(3) + u_4 * u_n_array(4);
else
    u_n_equation = 0;
end



u = e_n_equation + u_n_equation;

e_3 = e_2;
e_2=e_1;
e_1=e_0;

u_4 = u_3;
u_3 = u_2;
u_2 = u_1;

u_1=u;

end

== matlab function Discrete_Model/Discrete PI - Lead Controller With AW/Integrator2 ==
  settings: updateMethod=DISCRETE  sampleTime=T_sample
  data: e_0 input; u output; discrete_array input
function u = Controller(e_0, discrete_array)
persistent u_1 e_1 e_2 e_3 e_4 u_2 u_3 u_4 ;

coder.extrinsic('evalin', 'assignin') %% this allows access to T_sample
T = 0;
T = evalin('base','T_sample'); % Read value from workspace



%% discrete array input has the following format
%discrete_array(1) =  u_n FD array 
%discrete_array(2) =  e_n FD array 
%discrete_array(3) =  u_n BD array 
%discrete_array(4) =  e_n BD array 




%% With a FD controller
u_n_array = discrete_array(3, 1:end);
e_n_array = discrete_array(4, 1:end);











% Continuous controller : 
%tf_numerator = [1.203 3.6];
%tf_denomenator = [0.04812 1];




%Discrete output from program














if isempty(e_1)
    e_1 = 0;
end
if isempty(e_2)
    e_2 = 0;
end
if isempty(e_3)
    e_3 = 0;
end
if isempty(u_1)
    u_1 = 0;
end

if isempty(u_2)
    u_2 = 0;
end
if isempty(u_3)
    u_3 = 0;
end
if isempty(e_4)
    e_4 = 0;
end
if isempty(u_4)
    u_4 = 0;
end





e_n_length = length(e_n_array);
u_n_length = length(u_n_array); 

if e_n_length == 1
    e_n_equation = e_0 * e_n_array(1);
elseif e_n_length ==2
        e_n_equation = e_0 * e_n_array(1) + e_1 * e_n_array(2);
elseif e_n_length ==3
        e_n_equation = e_0 * e_n_array(1) + e_n_array(2) * e_1 + e_2 * e_n_array(3);
elseif e_n_length ==4
        e_n_equation = e_0 * e_n_array(1) + e_n_array(2) * e_1 + e_2 * e_n_array(3) + e_3 * e_n_array(4);
else
    e_n_equation = 0
end

if u_n_length == 1
        u_n_equation = u_1 * u_n_array(1);
elseif u_n_length == 2
        u_n_equation = u_1 * u_n_array(1) + u_2 * u_n_array(2);
elseif u_n_length ==3
        u_n_equation = u_1 * u_n_array(1) + u_n_array(2) * u_2 + u_3 * u_n_array(3);
elseif u_n_length ==4
        u_n_equation = u_1 * u_n_array(1) + u_n_array(2) * u_2 + u_3 * u_n_array(3) + u_4 * u_n_array(4);
else
    u_n_equation = 0;
end



u = e_n_equation + u_n_equation;

e_3 = e_2;
e_2=e_1;
e_1=e_0;

u_4 = u_3;
u_3 = u_2;
u_2 = u_1;

u_1=u;

end

== matlab function Discrete_Model/Cont//discrete controller No AW/Discrete Controller ==
  settings: updateMethod=DISCRETE  sampleTime=T_sample
  data: e_0 input; u output; discrete_array input
function u = Controller(e_0, discrete_array)
persistent u_1 e_1 e_2 e_3 e_4 u_2 u_3 u_4 ;

coder.extrinsic('evalin', 'assignin') %% this allows access to T_sample
T = 0;
T = evalin('base','T_sample'); % Read value from workspace



%% discrete array input has the following format
%discrete_array(1) =  u_n FD array 
%discrete_array(2) =  e_n FD array 
%discrete_array(3) =  u_n BD array 
%discrete_array(4) =  e_n BD array 



%% With a FD controller
u_n_array = discrete_array(1, 1:end);
e_n_array = discrete_array(2, 1:end);











% Continuous controller : 
%tf_numerator = [1.203 3.6];
%tf_denomenator = [0.04812 1];




%Discrete output from program














if isempty(e_1)
    e_1 = 0;
end
if isempty(e_2)
    e_2 = 0;
end
if isempty(e_3)
    e_3 = 0;
end
if isempty(u_1)
    u_1 = 0;
end

if isempty(u_2)
    u_2 = 0;
end
if isempty(u_3)
    u_3 = 0;
end
if isempty(e_4)
    e_4 = 0;
end
if isempty(u_4)
    u_4 = 0;
end





e_n_length = length(e_n_array);
u_n_length = length(u_n_array); 

if e_n_length == 1
    e_n_equation = e_0 * e_n_array(1);
elseif e_n_length ==2
        e_n_equation = e_0 * e_n_array(1) + e_1 * e_n_array(2);
elseif e_n_length ==3
        e_n_equation = e_0 * e_n_array(1) + e_n_array(2) * e_1 + e_2 * e_n_array(3);
elseif e_n_length ==4
        e_n_equation = e_0 * e_n_array(1) + e_n_array(2) * e_1 + e_2 * e_n_array(3) + e_3 * e_n_array(4);
else
    e_n_equation = 0
end

if u_n_length == 1
        u_n_equation = u_1 * u_n_array(1);
elseif u_n_length == 2
        u_n_equation = u_1 * u_n_array(1) + u_2 * u_n_array(2);
elseif u_n_length ==3
        u_n_equation = u_1 * u_n_array(1) + u_n_array(2) * u_2 + u_3 * u_n_array(3);
elseif u_n_length ==4
        u_n_equation = u_1 * u_n_array(1) + u_n_array(2) * u_2 + u_3 * u_n_array(3) + u_4 * u_n_array(4);
else
    u_n_equation = 0;
end



u = e_n_equation + u_n_equation;

%u = (1447209*e_2 + 1203000*T*u_1 - e_1*(30075000*T + 2894418) + e_0*(90000000*T^2 + 30075000*T + 1447209))/(1000*T*(25000*T + 1203));

e_3 = e_2;
e_2=e_1;
e_1=e_0;

u_4 = u_3;
u_3 = u_2;
u_2 = u_1;

u_1=u;

end
